simulink model "slxcases_R2025a"  (R2025a)
settings: Solver=VariableStepAuto
model workspace (MAT data in the model file):
  cfg.mode = 'fast'
  cfg.gain = 2
  flag = 1
  grid = [1  2  3; 4  5  6]
  inner = 7
  label = 'hello'
  names = {'alpha', 'beta'}
  span = 3
  tau = 0.25
undefined symbols (not defined in the file or in its folder): Ki, Kp
settings Model: DataDictionary=slxparams.sldd  Creator=weiwang  LastModifiedBy=weiwang
settings SFSimCC: SimGPUStackLimitPerThread=51200  SimGPUMallocThreshold=200
settings RTWCC: GPUStackLimitPerThread=51200  GPUMallocThreshold=200

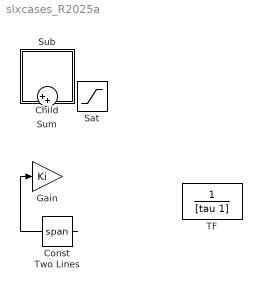
== system slxcases_R2025a ==
  Child : ModelReference  ModelNameDialog=slx_child  ModelReferenceVersion=1.1
  Const : Constant  Value=Kp
  Gain : Gain  Gain=Ki
  Sat : Saturate  UpperLimit=Inf  LowerLimit=-Inf
  Sub : Subsystem
  Sum : Sum  Inputs=|++
  TF : TransferFcn  Denominator=[tau 1]
  Two Lines : Constant  Value=span
  wires:
  Const/1 -> Gain/1

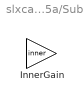
== system slxcases_R2025a/Sub ==
  InnerGain : Gain  Gain=inner
